simulink model "Count_Up_Down"  (R2021a)
settings: Solver=VariableStepAuto  StartTime=0.0  StopTime=10.0  RelTol=1e-3
settings Model: Creator=elkny  LastModifiedBy=elkny

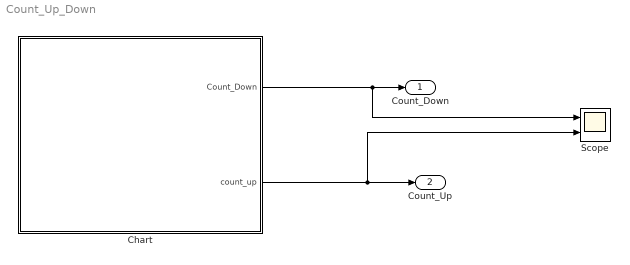
== system Count_Up_Down ==
  Chart : Stateflow chart  TreatAsAtomicUnit=on
  Scope : Scope  NumInputPorts=2
  Count_Down : Outport
  Count_Up : Outport  Port=2
  wires:
  Chart/2(count_up) -> Scope/2, Count_Up/1
  Chart/1(Count_Down) -> Scope/1, Count_Down/1

== stateflow chart Count_Up_Down/Chart ==
  state CountUP_Down
    entry:
    count_up=count_up+1;
    Count_Down=Count_Down-1;
  state Reset
    entry:
    count_up=0;
    Count_Down=10;
  (default) -> CountUP_Down
  CountUP_Down -> CountUP_Down [order 2] : {after(1,tick)}
  Reset -> CountUP_Down
  CountUP_Down -> Reset [order 1] : [count_up==10]
  data: Count_Down output =11; count_up output =-1
